simulink subsystem "MappedSteering"  (R2023b)
settings: Solver=VariableStepAuto  StartTime=0.0  StopTime=10.0  RelTol=1e-3
undefined symbols (not defined in the file): PlntSteerGearRatio
libraries: vehdynlibsteering x2
settings Model: ModifiedByFormat=The MathWorks, Inc.  Creator=The MathWorks, Inc.  LastModifiedBy=The MathWorks, Inc.

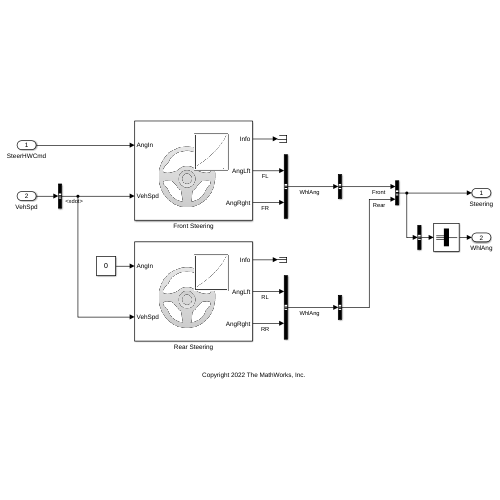
[thumbnail: Simulink's stored preview of the top-level diagram]
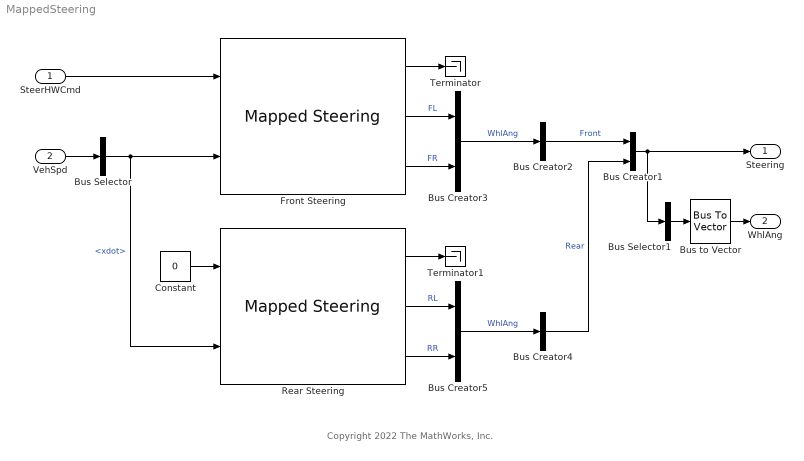
== system MappedSteering ==
  note: Copyright 2022 The MathWorks, Inc.
  SteerHWCmd : Inport
  VehSpd : Inport  Port=2
  Bus Creator1 : BusCreator  Inputs=2
  Bus Creator2 : BusCreator  Inputs=1
  Bus Creator3 : BusCreator  Inputs=2
  Bus Creator4 : BusCreator  Inputs=1
  Bus Creator5 : BusCreator  Inputs=2
  Bus Selector : BusSelector  OutputSignals=BdyFrm.Cg.Vel.xdot
  Bus Selector1 : BusSelector  OutputSignals=Front.WhlAng.FL,Front.WhlAng.FR,Rear.WhlAng.RL,Rear.WhlAng.RR  OutputAsBus=on
  Bus to Vector : BusToVector
  Constant : Constant  Value=0  SampleTime=-1
  Front Steering : vehdynlibsteering/Mapped Steering  SpdDpd=on  IndexType=Rack travel displacement  GrType=Constant  StrgAngBpts=[-1.5*pi 1.5*pi]  RackDispBpts=PlntSteerRackDispBpt  Gr=PlntSteerGearRatio  GrTbl=[9.87 9.87 7.16 7.16 9.87 9.87]*2*pi  WhlLftTbl=PlntSteerLftWhlAngTbl  WhlRghtTbl=PlntSteerRghtWhlAngTbl  VehSpdBpts=[-1 1]  SpdFctTbl=[1 1]  aMode=2
  Rear Steering : vehdynlibsteering/Mapped Steering  SpdDpd=on  IndexType=Rack travel displacement  GrType=Constant  StrgAngBpts=[-1.5*pi 1.5*pi]  RackDispBpts=PlntSteerRackDispBpt  Gr=PlntSteerGearRatio/10  GrTbl=[9.87 9.87 7.16 7.16 9.87 9.87]*2*pi  WhlLftTbl=PlntSteerLftWhlAngTbl  WhlRghtTbl=PlntSteerRghtWhlAngTbl  VehSpdBpts=[-1 1]  SpdFctTbl=[1 1]  aMode=2
  Terminator : Terminator
  Terminator1 : Terminator
  Steering : Outport
  WhlAng : Outport  Port=2  VectorParamsAs1DForOutWhenUnconnected=off
  wires:
  Bus Selector/1 -> Front Steering/2, Rear Steering/2  "<xdot>"
  VehSpd/1 -> Bus Selector/1
  SteerHWCmd/1 -> Front Steering/1
  Constant/1 -> Rear Steering/1
  Bus Creator3/1 -> Bus Creator2/1  "WhlAng"
  Bus Creator4/1 -> Bus Creator1/2  "Rear"
  Front Steering/2 -> Bus Creator3/1  "FL"
  Rear Steering/2 -> Bus Creator5/1  "RL"
  Rear Steering/3 -> Bus Creator5/2  "RR"
  Bus Creator2/1 -> Bus Creator1/1  "Front"
  Front Steering/3 -> Bus Creator3/2  "FR"
  Bus Creator5/1 -> Bus Creator4/1  "WhlAng"
  Front Steering/1 -> Terminator/1
  Rear Steering/1 -> Terminator1/1
  Bus Selector1/1 -> Bus to Vector/1
  Bus Creator1/1 -> Steering/1, Bus Selector1/1
  Bus to Vector/1 -> WhlAng/1
